simulink model "auto_irrigation_gr1"  (R2021a)
settings: Solver=VariableStepAuto  StartTime=0.0  StopTime=10  RelTol=1e-3
settings Model: Creator=user  LastModifiedBy=user

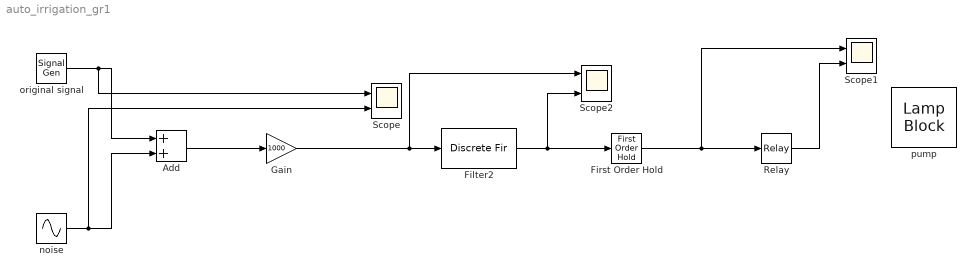
== system auto_irrigation_gr1 ==
  Add : Sum
  Filter2 : DiscreteFir  Tag=BlockMethodSubSystem  Coefficients=[0.00571446346349022485 0.0241000741155928122 0.0579779198981282828 0.0982019482360174389 0.126085225982440707 0.126085225982440707 0.0982019482360174389 0.0579779198981282828 0.0241000741155928122 0.00571446346349022485]  InputProcessing=Columns as channels (frame based)
  First Order Hold : FirstOrderHold  ErrorTolerance=inf
  Gain : Gain  Gain=1000
  Relay : Relay  OnSwitchValue=501  OffSwitchValue=500
  Scope : Scope  NumInputPorts=2
  Scope1 : Scope  NumInputPorts=2
  Scope2 : Scope  NumInputPorts=2
  noise : Sin  Amplitude=10  Frequency=110  SampleTime=0
  original signal : SignalGenerator  WaveForm=sawtooth  Amplitude=5  Frequency=5  Units=rad/sec
  pump : LampBlock
  wires:
  original signal/1 -> Scope/1, Add/1
  noise/1 -> Scope/2, Add/2
  Add/1 -> Gain/1
  Gain/1 -> Filter2/1, Scope2/1
  Filter2/1 -> Scope2/2, First Order Hold/1
  First Order Hold/1 -> Relay/1, Scope1/1
  Relay/1 -> Scope1/2
